simulink model "Noordergraaf_Rideout"  (R2022b)
settings: Solver=FixedStepAuto  StartTime=0.0  StopTime=stop_time  FixedStep=sample_time  RelTol=1e-3
InitFcn:
  | %init_fcn_noordergraaf_rideout
StopFcn:
  | %stop_fcn_noordergraaf_rideout
undefined symbols (not defined in the file or in its folder): C, Cep, Cev, Cla, Cpa, Cpp, Cpv, Cra, Csa, Csp, Csv, Dx, fcs0, fes0, fes1, fesmin, fev0, fev1, fmax, fmin, Gx, initx, ka, KElv, KErv, kes, kev, KRlv, KRrv, ksys, L, Lpa, Lsa, P0lv, P0rv, Pn, R, R_105, R_26, R_29, R_34, R_35, R_60, R_61, R_64, R_65, R_66, R_70, R_82, R_84, R_88, R_90, R_AT, R_SA, Rev, Rla, Rpa, Rpp, Rpv, Rra ... (+18)
libraries: ee_lib x421, fl_lib x87, nesl_utility x57, simulink x2
(part 2 of 9)

== system Noordergraaf_Rideout/ P_AA ==
  Electrical Reference3 : fl_lib/Electrical/Electrical Elements/Electrical Reference
  PS-Simulink Converter1 : nesl_utility/PS-Simulink Converter  PhysicalDomain=network_engine_domain  SubClassName=ps_output  LeftPortType=input  RightPortType=output  PseudoPeriodic=off  Frequencies=[]  VectorFormat=1-D array  Unit=1  AffineConversion=off
  To Workspace1 : ToWorkspace  VariableName=P_AA  SaveFormat=Timeseries  SampleTime=-1
  Voltage Sensor : fl_lib/Electrical/Electrical Sensors/Voltage Sensor
  Voltage Sensor1 : PMIOPort  Side=Left
  wires:
  PS-Simulink Converter1/1 -> To Workspace1/1
  connections:
  Electrical Reference3/LConn1 -- Voltage Sensor/RConn2
  PS-Simulink Converter1/LConn1 -- Voltage Sensor/RConn1
  Voltage Sensor/LConn1 -- Voltage Sensor1/RConn1

== system Noordergraaf_Rideout/ P_AAsc_in ==
  Electrical Reference3 : fl_lib/Electrical/Electrical Elements/Electrical Reference
  PS-Simulink Converter1 : nesl_utility/PS-Simulink Converter  PhysicalDomain=network_engine_domain  SubClassName=ps_output  LeftPortType=input  RightPortType=output  PseudoPeriodic=off  Frequencies=[]  VectorFormat=1-D array  Unit=1  AffineConversion=off
  To Workspace1 : ToWorkspace  VariableName=P_AAsc_in  SaveFormat=Timeseries  SampleTime=-1
  Voltage Sensor : fl_lib/Electrical/Electrical Sensors/Voltage Sensor
  Voltage Sensor1 : PMIOPort  Side=Left
  wires:
  PS-Simulink Converter1/1 -> To Workspace1/1
  connections:
  Voltage Sensor/LConn1 -- Voltage Sensor1/RConn1
  PS-Simulink Converter1/LConn1 -- Voltage Sensor/RConn1
  Electrical Reference3/LConn1 -- Voltage Sensor/RConn2

== system Noordergraaf_Rideout/ P_AAsc_out ==
  Electrical Reference3 : fl_lib/Electrical/Electrical Elements/Electrical Reference
  PS-Simulink Converter1 : nesl_utility/PS-Simulink Converter  PhysicalDomain=network_engine_domain  SubClassName=ps_output  LeftPortType=input  RightPortType=output  PseudoPeriodic=off  Frequencies=[]  VectorFormat=1-D array  Unit=1  AffineConversion=off
  To Workspace1 : ToWorkspace  VariableName=P_AAsc_out  SaveFormat=Timeseries  SampleTime=-1
  Voltage Sensor : fl_lib/Electrical/Electrical Sensors/Voltage Sensor
  Voltage Sensor1 : PMIOPort  Side=Left
  wires:
  PS-Simulink Converter1/1 -> To Workspace1/1
  connections:
  Voltage Sensor/LConn1 -- Voltage Sensor1/RConn1
  PS-Simulink Converter1/LConn1 -- Voltage Sensor/RConn1
  Electrical Reference3/LConn1 -- Voltage Sensor/RConn2

== system Noordergraaf_Rideout/ P_AbA ==
  Electrical Reference3 : fl_lib/Electrical/Electrical Elements/Electrical Reference
  PS-Simulink Converter1 : nesl_utility/PS-Simulink Converter  PhysicalDomain=network_engine_domain  SubClassName=ps_output  LeftPortType=input  RightPortType=output  PseudoPeriodic=off  Frequencies=[]  VectorFormat=1-D array  Unit=1  AffineConversion=off
  To Workspace1 : ToWorkspace  VariableName=P_AbA  SaveFormat=Timeseries  SampleTime=-1
  Voltage Sensor : fl_lib/Electrical/Electrical Sensors/Voltage Sensor
  Voltage Sensor1 : PMIOPort  Side=Left
  wires:
  PS-Simulink Converter1/1 -> To Workspace1/1
  connections:
  Electrical Reference3/LConn1 -- Voltage Sensor/RConn2
  PS-Simulink Converter1/LConn1 -- Voltage Sensor/RConn1
  Voltage Sensor/LConn1 -- Voltage Sensor1/RConn1

== system Noordergraaf_Rideout/ P_Aortic_Root ==
  Electrical Reference3 : fl_lib/Electrical/Electrical Elements/Electrical Reference
  PS-Simulink Converter1 : nesl_utility/PS-Simulink Converter  PhysicalDomain=network_engine_domain  SubClassName=ps_output  LeftPortType=input  RightPortType=output  PseudoPeriodic=off  Frequencies=[]  VectorFormat=1-D array  Unit=1  AffineConversion=off
  To Workspace1 : ToWorkspace  VariableName=P_Aortic_Root  SaveFormat=Timeseries  SampleTime=-1
  Voltage Sensor : fl_lib/Electrical/Electrical Sensors/Voltage Sensor
  Voltage Sensor1 : PMIOPort  Side=Left
  wires:
  PS-Simulink Converter1/1 -> To Workspace1/1
  connections:
  Electrical Reference3/LConn1 -- Voltage Sensor/RConn2
  PS-Simulink Converter1/LConn1 -- Voltage Sensor/RConn1
  Voltage Sensor/LConn1 -- Voltage Sensor1/RConn1

== system Noordergraaf_Rideout/ P_Axi ==
  Electrical Reference3 : fl_lib/Electrical/Electrical Elements/Electrical Reference
  PS-Simulink Converter1 : nesl_utility/PS-Simulink Converter  PhysicalDomain=network_engine_domain  SubClassName=ps_output  LeftPortType=input  RightPortType=output  PseudoPeriodic=off  Frequencies=[]  VectorFormat=1-D array  Unit=1  AffineConversion=off
  To Workspace1 : ToWorkspace  VariableName=P_Axi  SaveFormat=Timeseries  SampleTime=-1
  Voltage Sensor : fl_lib/Electrical/Electrical Sensors/Voltage Sensor
  Voltage Sensor1 : PMIOPort  Side=Left
  wires:
  PS-Simulink Converter1/1 -> To Workspace1/1
  connections:
  Electrical Reference3/LConn1 -- Voltage Sensor/RConn2
  PS-Simulink Converter1/LConn1 -- Voltage Sensor/RConn1
  Voltage Sensor/LConn1 -- Voltage Sensor1/RConn1

== system Noordergraaf_Rideout/ P_Brach ==
  Electrical Reference3 : fl_lib/Electrical/Electrical Elements/Electrical Reference
  PS-Simulink Converter1 : nesl_utility/PS-Simulink Converter  PhysicalDomain=network_engine_domain  SubClassName=ps_output  LeftPortType=input  RightPortType=output  PseudoPeriodic=off  Frequencies=[]  VectorFormat=1-D array  Unit=1  AffineConversion=off
  To Workspace1 : ToWorkspace  VariableName=P_Brach  SaveFormat=Timeseries  SampleTime=-1
  Voltage Sensor : fl_lib/Electrical/Electrical Sensors/Voltage Sensor
  Voltage Sensor1 : PMIOPort  Side=Right
  wires:
  PS-Simulink Converter1/1 -> To Workspace1/1
  connections:
  Electrical Reference3/LConn1 -- Voltage Sensor/RConn2
  PS-Simulink Converter1/LConn1 -- Voltage Sensor/RConn1
  Voltage Sensor/LConn1 -- Voltage Sensor1/RConn1

== system Noordergraaf_Rideout/ P_Carot ==
  Electrical Reference3 : fl_lib/Electrical/Electrical Elements/Electrical Reference
  PS-Simulink Converter1 : nesl_utility/PS-Simulink Converter  PhysicalDomain=network_engine_domain  SubClassName=ps_output  LeftPortType=input  RightPortType=output  PseudoPeriodic=off  Frequencies=[]  VectorFormat=1-D array  Unit=1  AffineConversion=off
  To Workspace1 : ToWorkspace  VariableName=P_Carot  SaveFormat=Timeseries  SampleTime=-1
  Voltage Sensor : fl_lib/Electrical/Electrical Sensors/Voltage Sensor
  Voltage Sensor1 : PMIOPort  Side=Right
  wires:
  PS-Simulink Converter1/1 -> To Workspace1/1
  connections:
  Electrical Reference3/LConn1 -- Voltage Sensor/RConn2
  PS-Simulink Converter1/LConn1 -- Voltage Sensor/RConn1
  Voltage Sensor/LConn1 -- Voltage Sensor1/RConn1

== system Noordergraaf_Rideout/ P_DescA ==
  Electrical Reference3 : fl_lib/Electrical/Electrical Elements/Electrical Reference
  PS-Simulink Converter1 : nesl_utility/PS-Simulink Converter  PhysicalDomain=network_engine_domain  SubClassName=ps_output  LeftPortType=input  RightPortType=output  PseudoPeriodic=off  Frequencies=[]  VectorFormat=1-D array  Unit=1  AffineConversion=off
  To Workspace1 : ToWorkspace  VariableName=P_DescA  SaveFormat=Timeseries  SampleTime=-1
  Voltage Sensor : fl_lib/Electrical/Electrical Sensors/Voltage Sensor
  Voltage Sensor1 : PMIOPort  Side=Left
  wires:
  PS-Simulink Converter1/1 -> To Workspace1/1
  connections:
  Voltage Sensor/LConn1 -- Voltage Sensor1/RConn1
  PS-Simulink Converter1/LConn1 -- Voltage Sensor/RConn1
  Electrical Reference3/LConn1 -- Voltage Sensor/RConn2

== system Noordergraaf_Rideout/ P_FA ==
  Electrical Reference3 : fl_lib/Electrical/Electrical Elements/Electrical Reference
  PS-Simulink Converter1 : nesl_utility/PS-Simulink Converter  PhysicalDomain=network_engine_domain  SubClassName=ps_output  LeftPortType=input  RightPortType=output  PseudoPeriodic=off  Frequencies=[]  VectorFormat=1-D array  Unit=1  AffineConversion=off
  To Workspace1 : ToWorkspace  VariableName=P_FA  SaveFormat=Timeseries  SampleTime=-1
  Voltage Sensor : fl_lib/Electrical/Electrical Sensors/Voltage Sensor
  Voltage Sensor1 : PMIOPort  Side=Right
  wires:
  PS-Simulink Converter1/1 -> To Workspace1/1
  connections:
  Electrical Reference3/LConn1 -- Voltage Sensor/RConn2
  PS-Simulink Converter1/LConn1 -- Voltage Sensor/RConn1
  Voltage Sensor/LConn1 -- Voltage Sensor1/RConn1

== system Noordergraaf_Rideout/ P_Iliac ==
  Electrical Reference3 : fl_lib/Electrical/Electrical Elements/Electrical Reference
  PS-Simulink Converter1 : nesl_utility/PS-Simulink Converter  PhysicalDomain=network_engine_domain  SubClassName=ps_output  LeftPortType=input  RightPortType=output  PseudoPeriodic=off  Frequencies=[]  VectorFormat=1-D array  Unit=1  AffineConversion=off
  To Workspace1 : ToWorkspace  VariableName=P_Iliac  SaveFormat=Timeseries  SampleTime=-1
  Voltage Sensor : fl_lib/Electrical/Electrical Sensors/Voltage Sensor
  Voltage Sensor1 : PMIOPort  Side=Left
  wires:
  PS-Simulink Converter1/1 -> To Workspace1/1
  connections:
  Electrical Reference3/LConn1 -- Voltage Sensor/RConn2
  PS-Simulink Converter1/LConn1 -- Voltage Sensor/RConn1
  Voltage Sensor/LConn1 -- Voltage Sensor1/RConn1

== system Noordergraaf_Rideout/ P_LV ==
  Electrical Reference3 : fl_lib/Electrical/Electrical Elements/Electrical Reference
  PS-Simulink Converter1 : nesl_utility/PS-Simulink Converter  PhysicalDomain=network_engine_domain  SubClassName=ps_output  LeftPortType=input  RightPortType=output  PseudoPeriodic=off  Frequencies=[]  VectorFormat=1-D array  Unit=1  AffineConversion=off
  To Workspace1 : ToWorkspace  VariableName=P_LV  SaveFormat=Timeseries  SampleTime=-1
  Voltage Sensor : fl_lib/Electrical/Electrical Sensors/Voltage Sensor
  Voltage Sensor1 : PMIOPort  Side=Left
  wires:
  PS-Simulink Converter1/1 -> To Workspace1/1
  connections:
  Voltage Sensor/LConn1 -- Voltage Sensor1/RConn1
  PS-Simulink Converter1/LConn1 -- Voltage Sensor/RConn1
  Electrical Reference3/LConn1 -- Voltage Sensor/RConn2

== system Noordergraaf_Rideout/ P_Po ==
  Electrical Reference3 : fl_lib/Electrical/Electrical Elements/Electrical Reference
  PS-Simulink Converter1 : nesl_utility/PS-Simulink Converter  PhysicalDomain=network_engine_domain  SubClassName=ps_output  LeftPortType=input  RightPortType=output  PseudoPeriodic=off  Frequencies=[]  VectorFormat=1-D array  Unit=1  AffineConversion=off
  To Workspace1 : ToWorkspace  VariableName=P_Po  SaveFormat=Timeseries  SampleTime=-1
  Voltage Sensor : fl_lib/Electrical/Electrical Sensors/Voltage Sensor
  Voltage Sensor1 : PMIOPort  Side=Right
  wires:
  PS-Simulink Converter1/1 -> To Workspace1/1
  connections:
  Electrical Reference3/LConn1 -- Voltage Sensor/RConn2
  PS-Simulink Converter1/LConn1 -- Voltage Sensor/RConn1
  Voltage Sensor/LConn1 -- Voltage Sensor1/RConn1

== system Noordergraaf_Rideout/ P_Rad ==
  Electrical Reference3 : fl_lib/Electrical/Electrical Elements/Electrical Reference
  PS-Simulink Converter1 : nesl_utility/PS-Simulink Converter  PhysicalDomain=network_engine_domain  SubClassName=ps_output  LeftPortType=input  RightPortType=output  PseudoPeriodic=off  Frequencies=[]  VectorFormat=1-D array  Unit=1  AffineConversion=off
  To Workspace1 : ToWorkspace  VariableName=P_Rad  SaveFormat=Timeseries  SampleTime=-1
  Voltage Sensor : fl_lib/Electrical/Electrical Sensors/Voltage Sensor
  Voltage Sensor1 : PMIOPort  Side=Right
  wires:
  PS-Simulink Converter1/1 -> To Workspace1/1
  connections:
  Electrical Reference3/LConn1 -- Voltage Sensor/RConn2
  PS-Simulink Converter1/LConn1 -- Voltage Sensor/RConn1
  Voltage Sensor/LConn1 -- Voltage Sensor1/RConn1

== system Noordergraaf_Rideout/ P_SubC ==
  Electrical Reference3 : fl_lib/Electrical/Electrical Elements/Electrical Reference
  PS-Simulink Converter1 : nesl_utility/PS-Simulink Converter  PhysicalDomain=network_engine_domain  SubClassName=ps_output  LeftPortType=input  RightPortType=output  PseudoPeriodic=off  Frequencies=[]  VectorFormat=1-D array  Unit=1  AffineConversion=off
  To Workspace1 : ToWorkspace  VariableName=P_SubC  SaveFormat=Timeseries  SampleTime=-1
  Voltage Sensor : fl_lib/Electrical/Electrical Sensors/Voltage Sensor
  Voltage Sensor1 : PMIOPort  Side=Left
  wires:
  PS-Simulink Converter1/1 -> To Workspace1/1
  connections:
  Electrical Reference3/LConn1 -- Voltage Sensor/RConn2
  PS-Simulink Converter1/LConn1 -- Voltage Sensor/RConn1
  Voltage Sensor/LConn1 -- Voltage Sensor1/RConn1

== system Noordergraaf_Rideout/ P_ThA ==
  Electrical Reference3 : fl_lib/Electrical/Electrical Elements/Electrical Reference
  PS-Simulink Converter1 : nesl_utility/PS-Simulink Converter  PhysicalDomain=network_engine_domain  SubClassName=ps_output  LeftPortType=input  RightPortType=output  PseudoPeriodic=off  Frequencies=[]  VectorFormat=1-D array  Unit=1  AffineConversion=off
  To Workspace1 : ToWorkspace  VariableName=P_ThA  SaveFormat=Timeseries  SampleTime=-1
  Voltage Sensor : fl_lib/Electrical/Electrical Sensors/Voltage Sensor
  Voltage Sensor1 : PMIOPort  Side=Left
  wires:
  PS-Simulink Converter1/1 -> To Workspace1/1
  connections:
  Electrical Reference3/LConn1 -- Voltage Sensor/RConn2
  PS-Simulink Converter1/LConn1 -- Voltage Sensor/RConn1
  Voltage Sensor/LConn1 -- Voltage Sensor1/RConn1

== system Noordergraaf_Rideout/ P_TibAnt ==
  Electrical Reference3 : fl_lib/Electrical/Electrical Elements/Electrical Reference
  PS-Simulink Converter1 : nesl_utility/PS-Simulink Converter  PhysicalDomain=network_engine_domain  SubClassName=ps_output  LeftPortType=input  RightPortType=output  PseudoPeriodic=off  Frequencies=[]  VectorFormat=1-D array  Unit=1  AffineConversion=off
  To Workspace1 : ToWorkspace  VariableName=P_TibAnt  SaveFormat=Timeseries  SampleTime=-1
  Voltage Sensor : fl_lib/Electrical/Electrical Sensors/Voltage Sensor
  Voltage Sensor1 : PMIOPort  Side=Left
  wires:
  PS-Simulink Converter1/1 -> To Workspace1/1
  connections:
  Electrical Reference3/LConn1 -- Voltage Sensor/RConn2
  PS-Simulink Converter1/LConn1 -- Voltage Sensor/RConn1
  Voltage Sensor/LConn1 -- Voltage Sensor1/RConn1

== system Noordergraaf_Rideout/ P_TibPost ==
  Electrical Reference3 : fl_lib/Electrical/Electrical Elements/Electrical Reference
  PS-Simulink Converter1 : nesl_utility/PS-Simulink Converter  PhysicalDomain=network_engine_domain  SubClassName=ps_output  LeftPortType=input  RightPortType=output  PseudoPeriodic=off  Frequencies=[]  VectorFormat=1-D array  Unit=1  AffineConversion=off
  To Workspace1 : ToWorkspace  VariableName=P_TibPost  SaveFormat=Timeseries  SampleTime=-1
  Voltage Sensor : fl_lib/Electrical/Electrical Sensors/Voltage Sensor
  Voltage Sensor1 : PMIOPort  Side=Right
  wires:
  PS-Simulink Converter1/1 -> To Workspace1/1
  connections:
  Electrical Reference3/LConn1 -- Voltage Sensor/RConn2
  PS-Simulink Converter1/LConn1 -- Voltage Sensor/RConn1
  Voltage Sensor/LConn1 -- Voltage Sensor1/RConn1

== system Noordergraaf_Rideout/ P_Uln ==
  Electrical Reference3 : fl_lib/Electrical/Electrical Elements/Electrical Reference
  PS-Simulink Converter1 : nesl_utility/PS-Simulink Converter  PhysicalDomain=network_engine_domain  SubClassName=ps_output  LeftPortType=input  RightPortType=output  PseudoPeriodic=off  Frequencies=[]  VectorFormat=1-D array  Unit=1  AffineConversion=off
  To Workspace1 : ToWorkspace  VariableName=P_Uln  SaveFormat=Timeseries  SampleTime=-1
  Voltage Sensor : fl_lib/Electrical/Electrical Sensors/Voltage Sensor
  Voltage Sensor1 : PMIOPort  Side=Left
  wires:
  PS-Simulink Converter1/1 -> To Workspace1/1
  connections:
  Electrical Reference3/LConn1 -- Voltage Sensor/RConn2
  PS-Simulink Converter1/LConn1 -- Voltage Sensor/RConn1
  Voltage Sensor/LConn1 -- Voltage Sensor1/RConn1

== system Noordergraaf_Rideout/ P_Vert ==
  Electrical Reference3 : fl_lib/Electrical/Electrical Elements/Electrical Reference
  PS-Simulink Converter1 : nesl_utility/PS-Simulink Converter  PhysicalDomain=network_engine_domain  SubClassName=ps_output  LeftPortType=input  RightPortType=output  PseudoPeriodic=off  Frequencies=[]  VectorFormat=1-D array  Unit=1  AffineConversion=off
  To Workspace1 : ToWorkspace  VariableName=P_Vert  SaveFormat=Timeseries  SampleTime=-1
  Voltage Sensor : fl_lib/Electrical/Electrical Sensors/Voltage Sensor
  Voltage Sensor1 : PMIOPort  Side=Right
  wires:
  PS-Simulink Converter1/1 -> To Workspace1/1
  connections:
  Electrical Reference3/LConn1 -- Voltage Sensor/RConn2
  PS-Simulink Converter1/LConn1 -- Voltage Sensor/RConn1
  Voltage Sensor/LConn1 -- Voltage Sensor1/RConn1

== system Noordergraaf_Rideout/ P_Vola ==
  Electrical Reference3 : fl_lib/Electrical/Electrical Elements/Electrical Reference
  PS-Simulink Converter1 : nesl_utility/PS-Simulink Converter  PhysicalDomain=network_engine_domain  SubClassName=ps_output  LeftPortType=input  RightPortType=output  PseudoPeriodic=off  Frequencies=[]  VectorFormat=1-D array  Unit=1  AffineConversion=off
  To Workspace1 : ToWorkspace  VariableName=P_Vola  SaveFormat=Timeseries  SampleTime=-1
  Voltage Sensor : fl_lib/Electrical/Electrical Sensors/Voltage Sensor
  Voltage Sensor1 : PMIOPort  Side=Right
  wires:
  PS-Simulink Converter1/1 -> To Workspace1/1
  connections:
  Electrical Reference3/LConn1 -- Voltage Sensor/RConn2
  PS-Simulink Converter1/LConn1 -- Voltage Sensor/RConn1
  Voltage Sensor/LConn1 -- Voltage Sensor1/RConn1

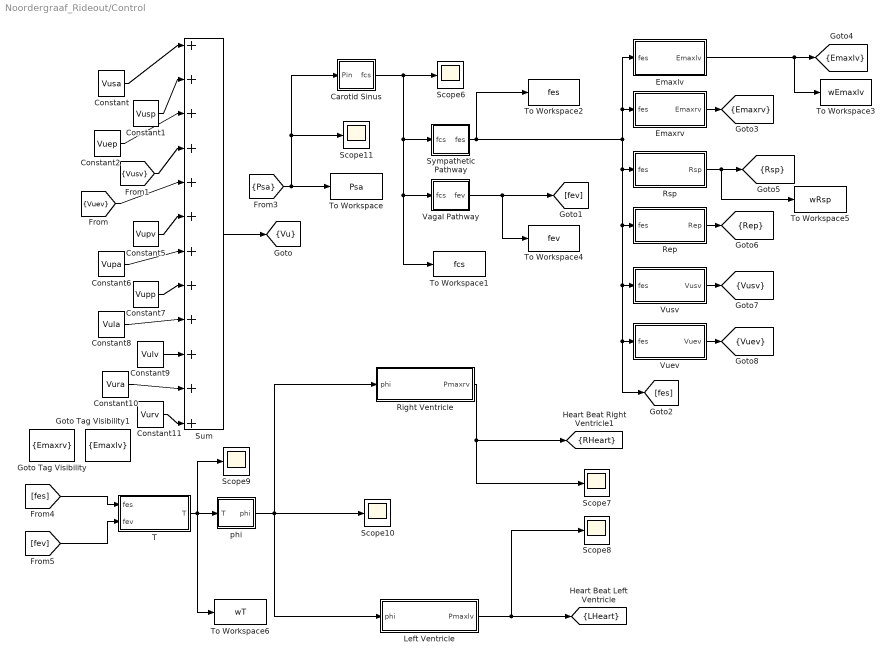
== system Noordergraaf_Rideout/Control ==
  Carotid Sinus : Subsystem
  Constant : Constant  Value=Vusa
  Constant1 : Constant  Value=Vusp
  Constant10 : Constant  Value=Vura
  Constant11 : Constant  Value=Vurv
  Constant2 : Constant  Value=Vuep
  Constant5 : Constant  Value=Vupv
  Constant6 : Constant  Value=Vupa
  Constant7 : Constant  Value=Vupp
  Constant8 : Constant  Value=Vula
  Constant9 : Constant  Value=Vulv
  Emaxlv : Subsystem
  Emaxrv : Subsystem
  Goto Tag Visibility : GotoTagVisibility  GotoTag=Emaxrv
  Goto Tag Visibility1 : GotoTagVisibility  GotoTag=Emaxlv
  Left Ventricle : Subsystem
  Rep : Subsystem
  Right Ventricle : Subsystem
  Rsp : Subsystem
  Scope{6..11} (6 alike) : Scope
  Sum : Sum  Inputs=|++++++++++++  SaturateOnIntegerOverflow=on
  Sympathetic Pathway : Subsystem
  T : Subsystem
  To Workspace : ToWorkspace  VariableName=Psa  SampleTime=-1
  To Workspace1 : ToWorkspace  VariableName=fcs  SampleTime=-1
  To Workspace2 : ToWorkspace  VariableName=fes  SampleTime=-1
  To Workspace3 : ToWorkspace  VariableName=wEmaxlv  SampleTime=-1
  To Workspace4 : ToWorkspace  VariableName=fev  SampleTime=-1
  To Workspace5 : ToWorkspace  VariableName=wRsp  SampleTime=-1
  To Workspace6 : ToWorkspace  VariableName=wT  SampleTime=-1
  Vagal Pathway : Subsystem
  Vuev : Subsystem
  Vusv : Subsystem
  phi : Subsystem
  tag scope: Emaxlv=scoped, Emaxrv=scoped, LHeart=scoped, RHeart=scoped, Rep=scoped, Rsp=scoped, Vu=scoped, Vuev=scoped, Vusv=scoped
  wires:
  Sum/1 -> [Vu]
  Constant/1 -> Sum/1
  Constant2/1 -> Sum/3
  Constant1/1 -> Sum/2
  [Vusv] -> Sum/4
  [Vuev] -> Sum/5
  Constant5/1 -> Sum/6
  Constant6/1 -> Sum/7
  Constant7/1 -> Sum/8
  Constant8/1 -> Sum/9
  Constant9/1 -> Sum/10
  Constant10/1 -> Sum/11
  Constant11/1 -> Sum/12
  Carotid Sinus/1(fcs) -> Scope6/1, Sympathetic Pathway/1(fcs), Vagal Pathway/1(fcs), To Workspace1/1
  [fes] -> T/1(fes)
  [fev] -> T/2(fev)
  phi/1(phi) -> Scope10/1, Right Ventricle/1(phi), Left Ventricle/1(phi)
  Right Ventricle/1(Pmaxrv) -> [RHeart], Scope7/1
  Left Ventricle/1(Pmaxlv) -> [LHeart], Scope8/1
  Sympathetic Pathway/1(fes) -> Emaxlv/1(fes), Emaxrv/1(fes), Rsp/1(fes), Rep/1(fes), Vusv/1(fes), Vuev/1(fes), [fes], To Workspace2/1
  Emaxrv/1(Emaxrv) -> [Emaxrv]
  Rep/1(Rep) -> [Rep]
  Vusv/1(Vusv) -> [Vusv]
  Vuev/1(Vuev) -> [Vuev]
  Vagal Pathway/1(fev) -> [fev], To Workspace4/1
  Rsp/1(Rsp) -> [Rsp], To Workspace5/1
  [Psa] -> To Workspace/1, Scope11/1, Carotid Sinus/1(Pin)
  T/1(T) -> Scope9/1, To Workspace6/1, phi/1(T)
  Emaxlv/1(Emaxlv) -> [Emaxlv], To Workspace3/1

== system Noordergraaf_Rideout/F_AT ==
  Current Sensor1 : fl_lib/Electrical/Electrical Sensors/Current Sensor
  PS-Simulink Converter1 : nesl_utility/PS-Simulink Converter  PhysicalDomain=network_engine_domain  SubClassName=ps_output  LeftPortType=input  RightPortType=output  PseudoPeriodic=off  Frequencies=[]  VectorFormat=1-D array  Unit=1  AffineConversion=off
  To Workspace : ToWorkspace  VariableName=F_AT  SaveFormat=Timeseries  SampleTime=-1
  I : PMIOPort  Side=Left
  O : PMIOPort  Port=2  Side=Right
  wires:
  PS-Simulink Converter1/1 -> To Workspace/1
  connections:
  Current Sensor1/LConn1 -- I/RConn1
  Current Sensor1/RConn1 -- PS-Simulink Converter1/LConn1
  Current Sensor1/RConn2 -- O/RConn1

== system Noordergraaf_Rideout/F_AbA ==
  Current Sensor : fl_lib/Electrical/Electrical Sensors/Current Sensor
  PS-Simulink Converter : nesl_utility/PS-Simulink Converter  PhysicalDomain=network_engine_domain  SubClassName=ps_output  LeftPortType=input  RightPortType=output  PseudoPeriodic=off  Frequencies=[]  VectorFormat=1-D array  Unit=1  AffineConversion=off
  To Workspace : ToWorkspace  VariableName=F_AbA  SaveFormat=Timeseries  SampleTime=-1
  O : PMIOPort  Side=Right
  I : PMIOPort  Port=2  Side=Left
  wires:
  PS-Simulink Converter/1 -> To Workspace/1
  connections:
  Current Sensor/RConn2 -- O/RConn1
  PS-Simulink Converter/LConn1 -- Current Sensor/RConn1
  I/RConn1 -- Current Sensor/LConn1

== system Noordergraaf_Rideout/F_AbA1 ==
  Current Sensor : fl_lib/Electrical/Electrical Sensors/Current Sensor
  PS-Simulink Converter : nesl_utility/PS-Simulink Converter  PhysicalDomain=network_engine_domain  SubClassName=ps_output  LeftPortType=input  RightPortType=output  PseudoPeriodic=off  Frequencies=[]  VectorFormat=1-D array  Unit=1  AffineConversion=off
  To Workspace : ToWorkspace  VariableName=F_AbA1  SaveFormat=Timeseries  SampleTime=-1
  O : PMIOPort  Side=Right
  I : PMIOPort  Port=2  Side=Left
  wires:
  PS-Simulink Converter/1 -> To Workspace/1
  connections:
  Current Sensor/RConn2 -- O/RConn1
  PS-Simulink Converter/LConn1 -- Current Sensor/RConn1
  I/RConn1 -- Current Sensor/LConn1

== system Noordergraaf_Rideout/F_Anon ==
  Current Sensor1 : fl_lib/Electrical/Electrical Sensors/Current Sensor
  PS-Simulink Converter1 : nesl_utility/PS-Simulink Converter  PhysicalDomain=network_engine_domain  SubClassName=ps_output  LeftPortType=input  RightPortType=output  PseudoPeriodic=off  Frequencies=[]  VectorFormat=1-D array  Unit=1  AffineConversion=off
  To Workspace : ToWorkspace  VariableName=F_Anon  SaveFormat=Timeseries  SampleTime=-1
  I : PMIOPort  Side=Left
  O : PMIOPort  Port=2  Side=Right
  wires:
  PS-Simulink Converter1/1 -> To Workspace/1
  connections:
  Current Sensor1/LConn1 -- I/RConn1
  Current Sensor1/RConn1 -- PS-Simulink Converter1/LConn1
  Current Sensor1/RConn2 -- O/RConn1

== system Noordergraaf_Rideout/F_Anon1 ==
  Current Sensor1 : fl_lib/Electrical/Electrical Sensors/Current Sensor
  PS-Simulink Converter1 : nesl_utility/PS-Simulink Converter  PhysicalDomain=network_engine_domain  SubClassName=ps_output  LeftPortType=input  RightPortType=output  PseudoPeriodic=off  Frequencies=[]  VectorFormat=1-D array  Unit=1  AffineConversion=off
  To Workspace : ToWorkspace  VariableName=F_Anon1  SaveFormat=Timeseries  SampleTime=-1
  I : PMIOPort  Side=Left
  O : PMIOPort  Port=2  Side=Right
  wires:
  PS-Simulink Converter1/1 -> To Workspace/1
  connections:
  Current Sensor1/LConn1 -- I/RConn1
  Current Sensor1/RConn1 -- PS-Simulink Converter1/LConn1
  Current Sensor1/RConn2 -- O/RConn1

== system Noordergraaf_Rideout/F_Arcus ==
  Current Sensor1 : fl_lib/Electrical/Electrical Sensors/Current Sensor
  PS-Simulink Converter1 : nesl_utility/PS-Simulink Converter  PhysicalDomain=network_engine_domain  SubClassName=ps_output  LeftPortType=input  RightPortType=output  PseudoPeriodic=off  Frequencies=[]  VectorFormat=1-D array  Unit=1  AffineConversion=off
  Scope : Scope
  To Workspace : ToWorkspace  VariableName=F_Arcus  SaveFormat=Timeseries  SampleTime=-1
  I : PMIOPort  Side=Left
  O : PMIOPort  Port=2  Side=Right
  wires:
  PS-Simulink Converter1/1 -> Scope/1, To Workspace/1
  connections:
  Current Sensor1/LConn1 -- I/RConn1
  Current Sensor1/RConn1 -- PS-Simulink Converter1/LConn1
  Current Sensor1/RConn2 -- O/RConn1

== system Noordergraaf_Rideout/F_Arcus2 ==
  Current Sensor1 : fl_lib/Electrical/Electrical Sensors/Current Sensor
  PS-Simulink Converter1 : nesl_utility/PS-Simulink Converter  PhysicalDomain=network_engine_domain  SubClassName=ps_output  LeftPortType=input  RightPortType=output  PseudoPeriodic=off  Frequencies=[]  VectorFormat=1-D array  Unit=1  AffineConversion=off
  Scope : Scope
  To Workspace : ToWorkspace  VariableName=F_Arcus2  SaveFormat=Timeseries  SampleTime=-1
  I : PMIOPort  Side=Left
  O : PMIOPort  Port=2  Side=Right
  wires:
  PS-Simulink Converter1/1 -> Scope/1, To Workspace/1
  connections:
  Current Sensor1/LConn1 -- I/RConn1
  Current Sensor1/RConn1 -- PS-Simulink Converter1/LConn1
  Current Sensor1/RConn2 -- O/RConn1

== system Noordergraaf_Rideout/F_Arcus3 ==
  Current Sensor1 : fl_lib/Electrical/Electrical Sensors/Current Sensor
  PS-Simulink Converter1 : nesl_utility/PS-Simulink Converter  PhysicalDomain=network_engine_domain  SubClassName=ps_output  LeftPortType=input  RightPortType=output  PseudoPeriodic=off  Frequencies=[]  VectorFormat=1-D array  Unit=1  AffineConversion=off
  Scope : Scope
  To Workspace : ToWorkspace  VariableName=F_Arcus3  SaveFormat=Timeseries  SampleTime=-1
  I : PMIOPort  Side=Left
  O : PMIOPort  Port=2  Side=Right
  wires:
  PS-Simulink Converter1/1 -> Scope/1, To Workspace/1
  connections:
  Current Sensor1/LConn1 -- I/RConn1
  Current Sensor1/RConn1 -- PS-Simulink Converter1/LConn1
  Current Sensor1/RConn2 -- O/RConn1

== system Noordergraaf_Rideout/F_Arcus4 ==
  Current Sensor1 : fl_lib/Electrical/Electrical Sensors/Current Sensor
  PS-Simulink Converter1 : nesl_utility/PS-Simulink Converter  PhysicalDomain=network_engine_domain  SubClassName=ps_output  LeftPortType=input  RightPortType=output  PseudoPeriodic=off  Frequencies=[]  VectorFormat=1-D array  Unit=1  AffineConversion=off
  Scope : Scope
  To Workspace : ToWorkspace  VariableName=F_Arcus4  SaveFormat=Timeseries  SampleTime=-1
  I : PMIOPort  Side=Left
  O : PMIOPort  Port=2  Side=Right
  wires:
  PS-Simulink Converter1/1 -> Scope/1, To Workspace/1
  connections:
  Current Sensor1/LConn1 -- I/RConn1
  Current Sensor1/RConn1 -- PS-Simulink Converter1/LConn1
  Current Sensor1/RConn2 -- O/RConn1

== system Noordergraaf_Rideout/F_Brach ==
  Current Sensor1 : fl_lib/Electrical/Electrical Sensors/Current Sensor
  PS-Simulink Converter1 : nesl_utility/PS-Simulink Converter  PhysicalDomain=network_engine_domain  SubClassName=ps_output  LeftPortType=input  RightPortType=output  PseudoPeriodic=off  Frequencies=[]  VectorFormat=1-D array  Unit=1  AffineConversion=off
  Scope : Scope
  To Workspace : ToWorkspace  VariableName=F_Brach  SaveFormat=Timeseries  SampleTime=-1
  I : PMIOPort  Side=Left
  O : PMIOPort  Port=2  Side=Right
  wires:
  PS-Simulink Converter1/1 -> Scope/1, To Workspace/1
  connections:
  Current Sensor1/LConn1 -- I/RConn1
  Current Sensor1/RConn1 -- PS-Simulink Converter1/LConn1
  Current Sensor1/RConn2 -- O/RConn1

== system Noordergraaf_Rideout/F_Brach1 ==
  Current Sensor1 : fl_lib/Electrical/Electrical Sensors/Current Sensor
  PS-Simulink Converter1 : nesl_utility/PS-Simulink Converter  PhysicalDomain=network_engine_domain  SubClassName=ps_output  LeftPortType=input  RightPortType=output  PseudoPeriodic=off  Frequencies=[]  VectorFormat=1-D array  Unit=1  AffineConversion=off
  Scope : Scope
  To Workspace : ToWorkspace  VariableName=F_Brach1  SaveFormat=Timeseries  SampleTime=-1
  I : PMIOPort  Side=Left
  O : PMIOPort  Port=2  Side=Right
  wires:
  PS-Simulink Converter1/1 -> Scope/1, To Workspace/1
  connections:
  Current Sensor1/LConn1 -- I/RConn1
  Current Sensor1/RConn1 -- PS-Simulink Converter1/LConn1
  Current Sensor1/RConn2 -- O/RConn1

== system Noordergraaf_Rideout/F_Coel ==
  Current Sensor1 : fl_lib/Electrical/Electrical Sensors/Current Sensor
  PS-Simulink Converter1 : nesl_utility/PS-Simulink Converter  PhysicalDomain=network_engine_domain  SubClassName=ps_output  LeftPortType=input  RightPortType=output  PseudoPeriodic=off  Frequencies=[]  VectorFormat=1-D array  Unit=1  AffineConversion=off
  To Workspace : ToWorkspace  VariableName=F_Coel  SaveFormat=Timeseries  SampleTime=-1
  I : PMIOPort  Side=Left
  O : PMIOPort  Port=2  Side=Right
  wires:
  PS-Simulink Converter1/1 -> To Workspace/1
  connections:
  Current Sensor1/LConn1 -- I/RConn1
  Current Sensor1/RConn1 -- PS-Simulink Converter1/LConn1
  Current Sensor1/RConn2 -- O/RConn1

== system Noordergraaf_Rideout/F_Fem ==
  Current Sensor1 : fl_lib/Electrical/Electrical Sensors/Current Sensor
  PS-Simulink Converter1 : nesl_utility/PS-Simulink Converter  PhysicalDomain=network_engine_domain  SubClassName=ps_output  LeftPortType=input  RightPortType=output  PseudoPeriodic=off  Frequencies=[]  VectorFormat=1-D array  Unit=1  AffineConversion=off
  Scope : Scope
  To Workspace : ToWorkspace  VariableName=F_Fem  SaveFormat=Timeseries  SampleTime=-1
  I : PMIOPort  Side=Left
  O : PMIOPort  Port=2  Side=Right
  wires:
  PS-Simulink Converter1/1 -> Scope/1, To Workspace/1
  connections:
  Current Sensor1/LConn1 -- I/RConn1
  Current Sensor1/RConn1 -- PS-Simulink Converter1/LConn1
  Current Sensor1/RConn2 -- O/RConn1

== system Noordergraaf_Rideout/F_Fem1 ==
  Current Sensor1 : fl_lib/Electrical/Electrical Sensors/Current Sensor
  PS-Simulink Converter1 : nesl_utility/PS-Simulink Converter  PhysicalDomain=network_engine_domain  SubClassName=ps_output  LeftPortType=input  RightPortType=output  PseudoPeriodic=off  Frequencies=[]  VectorFormat=1-D array  Unit=1  AffineConversion=off
  Scope : Scope
  To Workspace : ToWorkspace  VariableName=F_Fem1  SaveFormat=Timeseries  SampleTime=-1
  I : PMIOPort  Side=Left
  O : PMIOPort  Port=2  Side=Right
  wires:
  PS-Simulink Converter1/1 -> Scope/1, To Workspace/1
  connections:
  Current Sensor1/LConn1 -- I/RConn1
  Current Sensor1/RConn1 -- PS-Simulink Converter1/LConn1
  Current Sensor1/RConn2 -- O/RConn1

== system Noordergraaf_Rideout/F_Hep ==
  Current Sensor : fl_lib/Electrical/Electrical Sensors/Current Sensor
  PS-Simulink Converter : nesl_utility/PS-Simulink Converter  PhysicalDomain=network_engine_domain  SubClassName=ps_output  LeftPortType=input  RightPortType=output  PseudoPeriodic=off  Frequencies=[]  VectorFormat=1-D array  Unit=1  AffineConversion=off
  To Workspace : ToWorkspace  VariableName=F_Hep  SaveFormat=Timeseries  SampleTime=-1
  O : PMIOPort  Side=Right
  I : PMIOPort  Port=2  Side=Left
  wires:
  PS-Simulink Converter/1 -> To Workspace/1
  connections:
  Current Sensor/RConn2 -- O/RConn1
  PS-Simulink Converter/LConn1 -- Current Sensor/RConn1
  I/RConn1 -- Current Sensor/LConn1

== system Noordergraaf_Rideout/F_LV ==
  Current Sensor1 : fl_lib/Electrical/Electrical Sensors/Current Sensor
  PS-Simulink Converter1 : nesl_utility/PS-Simulink Converter  PhysicalDomain=network_engine_domain  SubClassName=ps_output  LeftPortType=input  RightPortType=output  PseudoPeriodic=off  Frequencies=[]  VectorFormat=1-D array  Unit=1  AffineConversion=off
  To Workspace : ToWorkspace  VariableName=F_LV  SaveFormat=Timeseries  SampleTime=-1
  I : PMIOPort  Side=Left
  O : PMIOPort  Port=2  Side=Right
  wires:
  PS-Simulink Converter1/1 -> To Workspace/1
  connections:
  Current Sensor1/LConn1 -- I/RConn1
  Current Sensor1/RConn1 -- PS-Simulink Converter1/LConn1
  Current Sensor1/RConn2 -- O/RConn1

== system Noordergraaf_Rideout/F_LegL ==
  Current Sensor1 : fl_lib/Electrical/Electrical Sensors/Current Sensor
  PS-Simulink Converter1 : nesl_utility/PS-Simulink Converter  PhysicalDomain=network_engine_domain  SubClassName=ps_output  LeftPortType=input  RightPortType=output  PseudoPeriodic=off  Frequencies=[]  VectorFormat=1-D array  Unit=1  AffineConversion=off
  Scope : Scope
  To Workspace : ToWorkspace  VariableName=F_LegL  SaveFormat=Timeseries  SampleTime=-1
  I : PMIOPort  Side=Left
  O : PMIOPort  Port=2  Side=Right
  wires:
  PS-Simulink Converter1/1 -> Scope/1, To Workspace/1
  connections:
  Current Sensor1/LConn1 -- I/RConn1
  Current Sensor1/RConn1 -- PS-Simulink Converter1/LConn1
  Current Sensor1/RConn2 -- O/RConn1

== system Noordergraaf_Rideout/F_LegR ==
  Current Sensor1 : fl_lib/Electrical/Electrical Sensors/Current Sensor
  PS-Simulink Converter1 : nesl_utility/PS-Simulink Converter  PhysicalDomain=network_engine_domain  SubClassName=ps_output  LeftPortType=input  RightPortType=output  PseudoPeriodic=off  Frequencies=[]  VectorFormat=1-D array  Unit=1  AffineConversion=off
  To Workspace : ToWorkspace  VariableName=F_LegR  SaveFormat=Timeseries  SampleTime=-1
  I : PMIOPort  Side=Left
  O : PMIOPort  Port=2  Side=Right
  wires:
  PS-Simulink Converter1/1 -> To Workspace/1
  connections:
  Current Sensor1/LConn1 -- I/RConn1
  Current Sensor1/RConn1 -- PS-Simulink Converter1/LConn1
  Current Sensor1/RConn2 -- O/RConn1

== system Noordergraaf_Rideout/F_Lien ==
  Current Sensor1 : fl_lib/Electrical/Electrical Sensors/Current Sensor
  PS-Simulink Converter1 : nesl_utility/PS-Simulink Converter  PhysicalDomain=network_engine_domain  SubClassName=ps_output  LeftPortType=input  RightPortType=output  PseudoPeriodic=off  Frequencies=[]  VectorFormat=1-D array  Unit=1  AffineConversion=off
  To Workspace : ToWorkspace  VariableName=F_Lien  SaveFormat=Timeseries  SampleTime=-1
  I : PMIOPort  Side=Left
  O : PMIOPort  Port=2  Side=Right
  wires:
  PS-Simulink Converter1/1 -> To Workspace/1
  connections:
  Current Sensor1/LConn1 -- I/RConn1
  Current Sensor1/RConn1 -- PS-Simulink Converter1/LConn1
  Current Sensor1/RConn2 -- O/RConn1

== system Noordergraaf_Rideout/F_MesI ==
  Current Sensor : fl_lib/Electrical/Electrical Sensors/Current Sensor
  PS-Simulink Converter : nesl_utility/PS-Simulink Converter  PhysicalDomain=network_engine_domain  SubClassName=ps_output  LeftPortType=input  RightPortType=output  PseudoPeriodic=off  Frequencies=[]  VectorFormat=1-D array  Unit=1  AffineConversion=off
  To Workspace : ToWorkspace  VariableName=F_MesI  SaveFormat=Timeseries  SampleTime=-1
  O : PMIOPort  Side=Right
  I : PMIOPort  Port=2  Side=Left
  wires:
  PS-Simulink Converter/1 -> To Workspace/1
  connections:
  Current Sensor/RConn2 -- O/RConn1
  PS-Simulink Converter/LConn1 -- Current Sensor/RConn1
  I/RConn1 -- Current Sensor/LConn1

== system Noordergraaf_Rideout/F_MesS ==
  Current Sensor1 : fl_lib/Electrical/Electrical Sensors/Current Sensor
  PS-Simulink Converter1 : nesl_utility/PS-Simulink Converter  PhysicalDomain=network_engine_domain  SubClassName=ps_output  LeftPortType=input  RightPortType=output  PseudoPeriodic=off  Frequencies=[]  VectorFormat=1-D array  Unit=1  AffineConversion=off
  To Workspace : ToWorkspace  VariableName=F_MesS  SaveFormat=Timeseries  SampleTime=-1
  I : PMIOPort  Side=Left
  O : PMIOPort  Port=2  Side=Right
  wires:
  PS-Simulink Converter1/1 -> To Workspace/1
  connections:
  Current Sensor1/LConn1 -- I/RConn1
  Current Sensor1/RConn1 -- PS-Simulink Converter1/LConn1
  Current Sensor1/RConn2 -- O/RConn1

== system Noordergraaf_Rideout/F_Po ==
  Current Sensor1 : fl_lib/Electrical/Electrical Sensors/Current Sensor
  PS-Simulink Converter1 : nesl_utility/PS-Simulink Converter  PhysicalDomain=network_engine_domain  SubClassName=ps_output  LeftPortType=input  RightPortType=output  PseudoPeriodic=off  Frequencies=[]  VectorFormat=1-D array  Unit=1  AffineConversion=off
  Scope : Scope
  To Workspace : ToWorkspace  VariableName=F_Po  SaveFormat=Timeseries  SampleTime=-1
  I : PMIOPort  Side=Left
  O : PMIOPort  Port=2  Side=Right
  wires:
  PS-Simulink Converter1/1 -> Scope/1, To Workspace/1
  connections:
  Current Sensor1/LConn1 -- I/RConn1
  Current Sensor1/RConn1 -- PS-Simulink Converter1/LConn1
  Current Sensor1/RConn2 -- O/RConn1

== system Noordergraaf_Rideout/F_Po1 ==
  Current Sensor1 : fl_lib/Electrical/Electrical Sensors/Current Sensor
  PS-Simulink Converter1 : nesl_utility/PS-Simulink Converter  PhysicalDomain=network_engine_domain  SubClassName=ps_output  LeftPortType=input  RightPortType=output  PseudoPeriodic=off  Frequencies=[]  VectorFormat=1-D array  Unit=1  AffineConversion=off
  Scope : Scope
  To Workspace : ToWorkspace  VariableName=F_Po1  SaveFormat=Timeseries  SampleTime=-1
  I : PMIOPort  Side=Left
  O : PMIOPort  Port=2  Side=Right
  wires:
  PS-Simulink Converter1/1 -> Scope/1, To Workspace/1
  connections:
  Current Sensor1/LConn1 -- I/RConn1
  Current Sensor1/RConn1 -- PS-Simulink Converter1/LConn1
  Current Sensor1/RConn2 -- O/RConn1

== system Noordergraaf_Rideout/F_Rena ==
  Current Sensor1 : fl_lib/Electrical/Electrical Sensors/Current Sensor
  PS-Simulink Converter1 : nesl_utility/PS-Simulink Converter  PhysicalDomain=network_engine_domain  SubClassName=ps_output  LeftPortType=input  RightPortType=output  PseudoPeriodic=off  Frequencies=[]  VectorFormat=1-D array  Unit=1  AffineConversion=off
  Scope : Scope
  To Workspace : ToWorkspace  VariableName=F_Rena  SaveFormat=Timeseries  SampleTime=-1
  I : PMIOPort  Side=Left
  O : PMIOPort  Port=2  Side=Right
  wires:
  PS-Simulink Converter1/1 -> Scope/1, To Workspace/1
  connections:
  Current Sensor1/LConn1 -- I/RConn1
  Current Sensor1/RConn1 -- PS-Simulink Converter1/LConn1
  Current Sensor1/RConn2 -- O/RConn1

== system Noordergraaf_Rideout/F_Rend ==
  Current Sensor1 : fl_lib/Electrical/Electrical Sensors/Current Sensor
  PS-Simulink Converter1 : nesl_utility/PS-Simulink Converter  PhysicalDomain=network_engine_domain  SubClassName=ps_output  LeftPortType=input  RightPortType=output  PseudoPeriodic=off  Frequencies=[]  VectorFormat=1-D array  Unit=1  AffineConversion=off
  To Workspace : ToWorkspace  VariableName=F_Rend  SaveFormat=Timeseries  SampleTime=-1
  I : PMIOPort  Side=Left
  O : PMIOPort  Port=2  Side=Right
  wires:
  PS-Simulink Converter1/1 -> To Workspace/1
  connections:
  Current Sensor1/LConn1 -- I/RConn1
  Current Sensor1/RConn1 -- PS-Simulink Converter1/LConn1
  Current Sensor1/RConn2 -- O/RConn1

== system Noordergraaf_Rideout/F_SubC ==
  Current Sensor1 : fl_lib/Electrical/Electrical Sensors/Current Sensor
  PS-Simulink Converter1 : nesl_utility/PS-Simulink Converter  PhysicalDomain=network_engine_domain  SubClassName=ps_output  LeftPortType=input  RightPortType=output  PseudoPeriodic=off  Frequencies=[]  VectorFormat=1-D array  Unit=1  AffineConversion=off
  Scope : Scope
  To Workspace : ToWorkspace  VariableName=F_SubC  SaveFormat=Timeseries  SampleTime=-1
  I : PMIOPort  Side=Left
  O : PMIOPort  Port=2  Side=Right
  wires:
  PS-Simulink Converter1/1 -> Scope/1, To Workspace/1
  connections:
  Current Sensor1/LConn1 -- I/RConn1
  Current Sensor1/RConn1 -- PS-Simulink Converter1/LConn1
  Current Sensor1/RConn2 -- O/RConn1

== system Noordergraaf_Rideout/F_SubC1 ==
  Current Sensor1 : fl_lib/Electrical/Electrical Sensors/Current Sensor
  PS-Simulink Converter1 : nesl_utility/PS-Simulink Converter  PhysicalDomain=network_engine_domain  SubClassName=ps_output  LeftPortType=input  RightPortType=output  PseudoPeriodic=off  Frequencies=[]  VectorFormat=1-D array  Unit=1  AffineConversion=off
  Scope : Scope
  To Workspace : ToWorkspace  VariableName=F_SubC1  SaveFormat=Timeseries  SampleTime=-1
  I : PMIOPort  Side=Left
  O : PMIOPort  Port=2  Side=Right
  wires:
  PS-Simulink Converter1/1 -> Scope/1, To Workspace/1
  connections:
  Current Sensor1/LConn1 -- I/RConn1
  Current Sensor1/RConn1 -- PS-Simulink Converter1/LConn1
  Current Sensor1/RConn2 -- O/RConn1

== system Noordergraaf_Rideout/F_ThA ==
  Current Sensor : fl_lib/Electrical/Electrical Sensors/Current Sensor
  PS-Simulink Converter : nesl_utility/PS-Simulink Converter  PhysicalDomain=network_engine_domain  SubClassName=ps_output  LeftPortType=input  RightPortType=output  PseudoPeriodic=off  Frequencies=[]  VectorFormat=1-D array  Unit=1  AffineConversion=off
  To Workspace : ToWorkspace  VariableName=F_ThA  SaveFormat=Timeseries  SampleTime=-1
  O : PMIOPort  Side=Right
  I : PMIOPort  Port=2  Side=Left
  wires:
  PS-Simulink Converter/1 -> To Workspace/1
  connections:
  Current Sensor/RConn2 -- O/RConn1
  PS-Simulink Converter/LConn1 -- Current Sensor/RConn1
  I/RConn1 -- Current Sensor/LConn1

== system Noordergraaf_Rideout/F_ThA1 ==
  Current Sensor : fl_lib/Electrical/Electrical Sensors/Current Sensor
  PS-Simulink Converter : nesl_utility/PS-Simulink Converter  PhysicalDomain=network_engine_domain  SubClassName=ps_output  LeftPortType=input  RightPortType=output  PseudoPeriodic=off  Frequencies=[]  VectorFormat=1-D array  Unit=1  AffineConversion=off
  To Workspace : ToWorkspace  VariableName=F_ThA1  SaveFormat=Timeseries  SampleTime=-1
  O : PMIOPort  Side=Right
  I : PMIOPort  Port=2  Side=Left
  wires:
  PS-Simulink Converter/1 -> To Workspace/1
  connections:
  Current Sensor/RConn2 -- O/RConn1
  PS-Simulink Converter/LConn1 -- Current Sensor/RConn1
  I/RConn1 -- Current Sensor/LConn1

== system Noordergraaf_Rideout/F_Uln ==
  Current Sensor1 : fl_lib/Electrical/Electrical Sensors/Current Sensor
  PS-Simulink Converter1 : nesl_utility/PS-Simulink Converter  PhysicalDomain=network_engine_domain  SubClassName=ps_output  LeftPortType=input  RightPortType=output  PseudoPeriodic=off  Frequencies=[]  VectorFormat=1-D array  Unit=1  AffineConversion=off
  Scope : Scope
  To Workspace : ToWorkspace  VariableName=F_Uln  SaveFormat=Timeseries  SampleTime=-1
  I : PMIOPort  Side=Left
  O : PMIOPort  Port=2  Side=Right
  wires:
  PS-Simulink Converter1/1 -> Scope/1, To Workspace/1
  connections:
  Current Sensor1/LConn1 -- I/RConn1
  Current Sensor1/RConn1 -- PS-Simulink Converter1/LConn1
  Current Sensor1/RConn2 -- O/RConn1

== system Noordergraaf_Rideout/F_Uln1 ==
  Current Sensor1 : fl_lib/Electrical/Electrical Sensors/Current Sensor
  PS-Simulink Converter1 : nesl_utility/PS-Simulink Converter  PhysicalDomain=network_engine_domain  SubClassName=ps_output  LeftPortType=input  RightPortType=output  PseudoPeriodic=off  Frequencies=[]  VectorFormat=1-D array  Unit=1  AffineConversion=off
  Scope : Scope
  To Workspace : ToWorkspace  VariableName=F_Uln1  SaveFormat=Timeseries  SampleTime=-1
  I : PMIOPort  Side=Left
  O : PMIOPort  Port=2  Side=Right
  wires:
  PS-Simulink Converter1/1 -> Scope/1, To Workspace/1
  connections:
  Current Sensor1/LConn1 -- I/RConn1
  Current Sensor1/RConn1 -- PS-Simulink Converter1/LConn1
  Current Sensor1/RConn2 -- O/RConn1

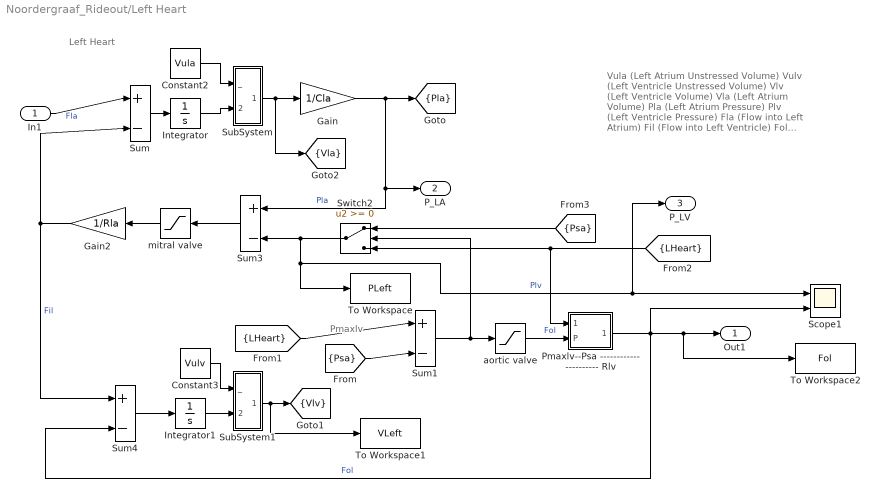
== system Noordergraaf_Rideout/Left Heart ==
  note: Left Heart
  note: Vula (Left Atrium Unstressed Volume)
      | Vulv (Left Ventricle Unstressed Volume)
      | Vlv (Left Ventricle Volume)
      | Vla (Left Atrium Volume)
      | Pla (Left Atrium Pressure)
      | Plv (Left Ventricle Pressure)
      | Fla (Flow into Left Atrium)
      | Fil (Flow into Left Ventricle)
      | Fol (Flow out of Left Ventricle)
      | LHeart (Left Ventricle Function)
  note: Pmaxlv
  In1 : Inport
  Constant2 : Constant  Value=Vula
  Constant3 : Constant  Value=Vulv
  Gain : Gain  Gain=1/Cla  SaturateOnIntegerOverflow=on
  Gain2 : Gain  Gain=1/Rla  SaturateOnIntegerOverflow=on
  Integrator : Integrator
  Integrator1 : Integrator
  Pmaxlv--Psa ---------------------- Rlv : Subsystem
  Scope1 : Scope  NumInputPorts=2
  SubSystem : Subsystem
  SubSystem1 : Subsystem
  Sum : Sum  Inputs=|+-  SaturateOnIntegerOverflow=on
  Sum1 : Sum  Inputs=|+-  SaturateOnIntegerOverflow=on
  Sum3 : Sum  Inputs=+-  SaturateOnIntegerOverflow=on
  Sum4 : Sum  Inputs=+-  SaturateOnIntegerOverflow=on
  Switch2 : Switch
  To Workspace : ToWorkspace  VariableName=PLeft  SampleTime=-1
  To Workspace1 : ToWorkspace  VariableName=VLeft  SampleTime=-1
  To Workspace2 : ToWorkspace  VariableName=Fol  SampleTime=-1
  aortic valve : Saturate  UpperLimit=inf  LowerLimit=0
  mitral valve : Saturate  UpperLimit=inf  LowerLimit=0
  Out1 : Outport
  P_LA : Outport  Port=2
  P_LV : Outport  Port=3
  tag scope: Pla=scoped, Vla=scoped, Vlv=scoped
  wires:
  In1/1 -> Sum/1  "Fla"
  Sum/1 -> Integrator/1
  [Psa] -> Sum1/2
  Gain/1 -> [Pla], P_LA/1, Sum3/1  "Pla"
  Sum4/1 -> Integrator1/1
  Gain2/1 -> Sum/2, Sum4/1  "Fil"
  Pmaxlv--Psa ---------------------- Rlv/1(Flow) -> Scope1/2, To Workspace2/1, Out1/1, Sum4/2  "Fol"
  Constant2/1 -> SubSystem/1(_)
  Constant3/1 -> SubSystem1/1(_)
  SubSystem/1(Out) -> Gain/1, [Vla]
  [LHeart] -> Sum1/1
  Sum1/1 -> aortic valve/1, Switch2/2
  [Psa] -> Switch2/1
  mitral valve/1 -> Gain2/1
  aortic valve/1 -> Pmaxlv--Psa ---------------------- Rlv/2(P)  "Fol"
  Switch2/1 -> Sum3/2, To Workspace/1, P_LV/1, Scope1/1  "Plv"
  Integrator1/1 -> SubSystem1/2(+)
  Sum3/1 -> mitral valve/1
  Integrator/1 -> SubSystem/2(+)
  [LHeart] -> Switch2/3, Pmaxlv--Psa ---------------------- Rlv/1(Pmax)
  SubSystem1/1(Out) -> [Vlv], To Workspace1/1

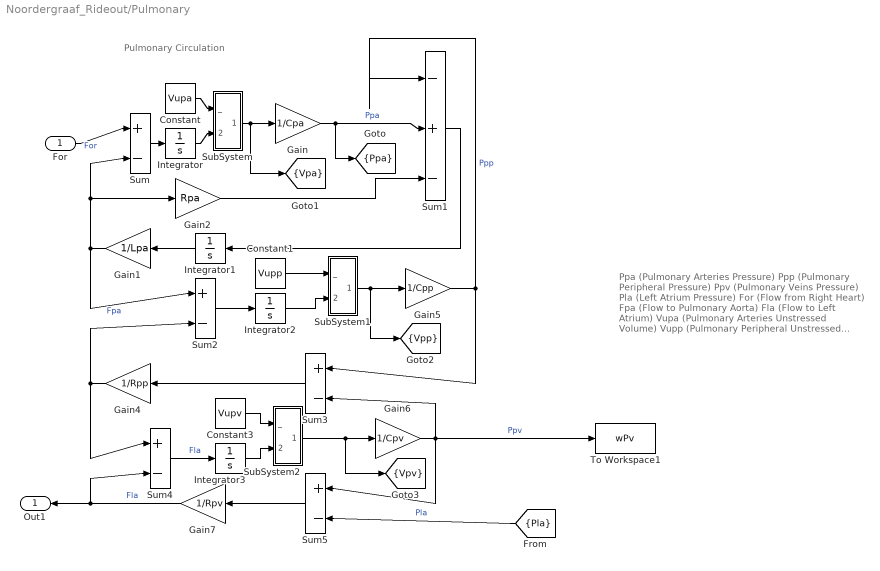
== system Noordergraaf_Rideout/Pulmonary ==
  note: Ppa (Pulmonary Arteries Pressure)
      | Ppp (Pulmonary Peripheral Pressure)
      | Ppv (Pulmonary Veins Pressure)
      | Pla (Left Atrium Pressure)
      | For (Flow from Right Heart)
      | Fpa (Flow to Pulmonary Aorta)
      | Fla (Flow to Left Atrium)
      | Vupa (Pulmonary Arteries Unstressed Volume)
      | Vupp (Pulmonary Peripheral Unstressed Volume)
      | Vupv (Pulmonary Veins Unstressed Volume)
  note: Pulmonary Circulation
  For : Inport
  Constant : Constant  Value=Vupa
  Constant1 : Constant  Value=Vupp
  Constant3 : Constant  Value=Vupv
  Gain : Gain  Gain=1/Cpa  SaturateOnIntegerOverflow=on
  Gain1 : Gain  Gain=1/Lpa  SaturateOnIntegerOverflow=on
  Gain2 : Gain  Gain=Rpa  SaturateOnIntegerOverflow=on
  Gain4 : Gain  Gain=1/Rpp  SaturateOnIntegerOverflow=on
  Gain5 : Gain  Gain=1/Cpp  SaturateOnIntegerOverflow=on
  Gain6 : Gain  Gain=1/Cpv  SaturateOnIntegerOverflow=on
  Gain7 : Gain  Gain=1/Rpv  SaturateOnIntegerOverflow=on
  Integrator : Integrator  InitialCondition=100
  Integrator1 : Integrator
  Integrator2 : Integrator  InitialCondition=100
  Integrator3 : Integrator
  SubSystem : Subsystem
  SubSystem1 : Subsystem
  SubSystem2 : Subsystem
  Sum{,2..5} (5 alike) : Sum  Inputs=|+-  SaturateOnIntegerOverflow=on
  Sum1 : Sum  Inputs=|-+-  SaturateOnIntegerOverflow=on
  To Workspace1 : ToWorkspace  VariableName=wPv  SampleTime=-1
  Out1 : Outport
  tag scope: Ppa=scoped, Vpa=scoped, Vpp=scoped, Vpv=scoped
  wires:
  For/1 -> Sum/1  "For"
  Sum/1 -> Integrator/1
  Integrator1/1 -> Gain1/1
  Sum1/1 -> Integrator1/1
  Gain2/1 -> Sum1/3
  Gain1/1 -> Sum/2, Gain2/1, Sum2/1  "Fpa"
  Sum2/1 -> Integrator2/1
  Gain5/1 -> Sum1/1, Sum3/1  "Ppp"
  Sum3/1 -> Gain4/1
  Gain4/1 -> Sum2/2, Sum4/1
  Sum5/1 -> Gain7/1
  Gain6/1 -> Sum3/2, Sum5/1, To Workspace1/1  "Ppv"
  [Pla] -> Sum5/2  "Pla"
  Sum4/1 -> Integrator3/1  "Fla"
  Gain/1 -> Sum1/2, [Ppa]  "Ppa"
  SubSystem/1(Out) -> Gain/1, [Vpa]
  SubSystem1/1(Out) -> Gain5/1, [Vpp]
  SubSystem2/1(Out) -> Gain6/1, [Vpv]
  Integrator/1 -> SubSystem/2(+)
  Constant/1 -> SubSystem/1(_)
  Constant1/1 -> SubSystem1/1(_)
  Integrator2/1 -> SubSystem1/2(+)
  Integrator3/1 -> SubSystem2/2(+)
  Gain7/1 -> Sum4/2, Out1/1  "Fla"
  Constant3/1 -> SubSystem2/1(_)
